simulink model "Sim2dot0"  (R2023b)
settings: Solver=VariableStepAuto  StartTime=0.0  StopTime=8  RelTol=1e-3
values from neighbouring files (symbols this model uses):
  cg_z = 0.335    [para_sim1dot4.mat]    (also in para_sim1dot5.mat; para_sim1dot6.mat = 0.215; para_sim1dot7.mat = 0.215)
  dt = 0.02    [para_sim1dot0.mat]    (also in para_sim1dot1.mat; para_sim1dot2.mat; para_sim1dot3.mat; para_sim1dot4.mat)
  F35thrust = [0 0.011 0.018 0.024 0.031 0.037 0.046 0.053 0.061 0.07 0.079 0.088 ... (170 elements, 85x2)]    [para_sim1dot3.mat]    (also in para_sim1dot4.mat; para_sim1dot5.mat; para_sim1dot6.mat; para_sim1dot7.mat)
  fin_drag_over_v2 = [-30 -25 -20 -15 -10 -5 0 5 10 15 20 25 ... (26 elements, 13x2)]    [para_sim1dot2.mat]    (also in para_sim1dot3.mat; para_sim1dot4.mat; para_sim1dot5.mat; para_sim1dot6.mat)
  fin_lift_over_v2 = [-30 -25 -20 -15 -10 -5 0 5 10 15 20 25 ... (26 elements, 13x2)]    [para_sim1dot2.mat]    (also in para_sim1dot3.mat; para_sim1dot4.mat; para_sim1dot5.mat; para_sim1dot6.mat)
  l_arm_moment = 0.5    [para_sim1dot2.mat]    (also in para_sim1dot3.mat; para_sim1dot4.mat = 0.3; para_sim1dot5.mat = 0.3; para_sim1dot6.mat = 0.175)
  mass = 1    [para_sim1dot0.mat]    (also in para_sim1dot1.mat; para_sim1dot2.mat = 0.6; para_sim1dot3.mat = 0.8; para_sim1dot4.mat = 0.8)
  max_fin_angle_deg = 30    [para_sim1dot0.mat]    (also in para_sim1dot1.mat; para_sim1dot2.mat; para_sim1dot3.mat; para_sim1dot4.mat = 20)
  r_arm_moment = 0.05    [para_sim1dot2.mat]    (also in para_sim1dot3.mat; para_sim1dot4.mat; para_sim1dot5.mat; para_sim1dot6.mat = 0.065)
  servo_slew_radps = 31.4    [para_sim1dot4.mat]    (also in para_sim1dot5.mat = 5.23; para_sim1dot6.mat = 5.23; para_sim1dot7.mat = 5.23)
libraries: simulink_extras x13, simulink x3, slpidlib x3, shared6dof x1, aerolibanim x1, matrix_library x1, aerolibanimutils x1
settings Model: Creator=Zian Liu  LastModifiedBy=Zian Liu

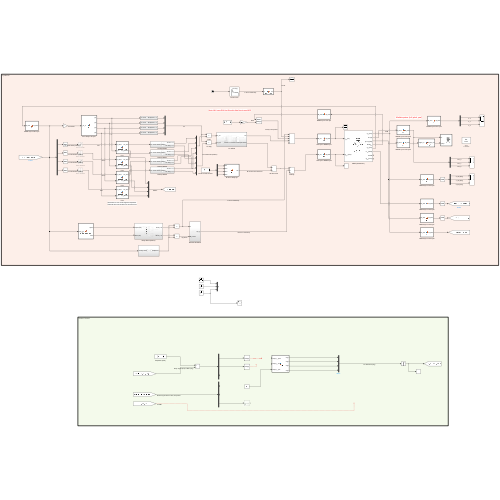
[thumbnail: Simulink's stored preview of the top-level diagram]
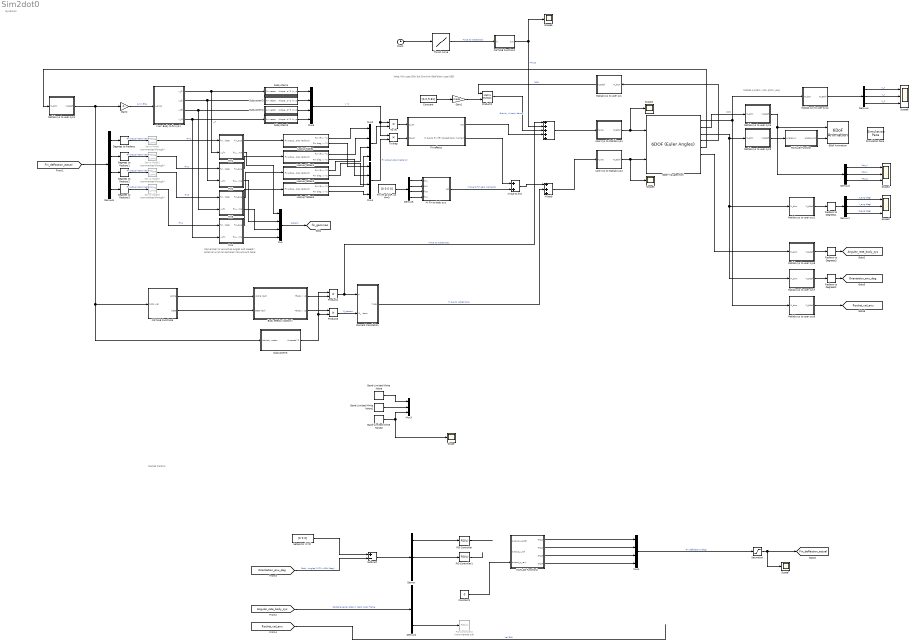
== system Sim2dot0 ==
  note: Dynamics
  note: Rocket Control
  note: Matlab system: [roll, pitch, yaw]
  note: Note: IMU uses ENU but Simulink 6dof block uses NED
  note: Remember to use actual angles and speeds!
      | External wind can be taken into account here!
  " " : Sum  Inputs=+++++
  6DOF (Quaternion) : shared6dof/6DOF (Euler Angles)  units=Metric (MKS)  mtype=Fixed  rep=Quaternion  xme_0=[0 0 0]  Vm_0=[0 0 0]  eul_0=[10*pi/180 0 0]  pm_0=[0 0 0]  mass_0=mass  mass_e=0.5  mass_f=2.0  inertia=diag([0.0301315, 0.0301315, 0.0004096])  inertia_e=eye(3)  inertia_f=2*eye(3)  k_quat=1.0  vre_flag=on  abi_flag=off  aMode=0  xme_statename=''  Vm_statename=''  eul_statename=''  quat_statename={'qr', 'qi', 'qj','qk'}  pm_statename=''  mass_statename=''
      settings: LibrarySourceBlock=aerolib6dof2/6DOF (Quaternion)
  6DoF Animation : aerolibanim/6DoF Animation  u1=[-100 100 -100 100 -300 300]  u2=0.1  u3=100  u4=[10000 0 0]  u5=Fly alongside  u6=[10000 0 0]  u7=0  u8=off
  Band-Limited White Noise : simulink/Sources/Band-Limited White Noise  Cov=[0.1]  Ts=0.01  seed=[23341]
  Band-Limited White Noise1 : simulink/Sources/Band-Limited White Noise  Cov=[0.1]  Ts=0.01  seed=[23342]
  Band-Limited White Noise2 : simulink/Sources/Band-Limited White Noise  Cov=[0.1]  Ts=0.01  seed=[23343]
  Body effects (bottom) : Subsystem
  Clock : Clock
  Constant : Constant  Value=[0,0,9.81]
  Constant1 : Constant  Value=0
  Degrees to Radians{,1..3} (4 alike) : simulink_extras/Transformations/Degrees to Radians
  Demux{,1..4} (5 alike) : Demux  Outputs=3
  Demux5 : Demux
  Demux6 : Demux
  Fin effects : Subsystem
  "Fin lift at CoP, so M=0" : Constant  Value=[0 0 0 0]
  Fin1 : MATLAB Function  TreatAsAtomicUnit=on
  Fin2 : MATLAB Function  TreatAsAtomicUnit=on
  Fin3 : MATLAB Function  TreatAsAtomicUnit=on
  Fin4 : MATLAB Function  TreatAsAtomicUnit=on
  Gain1 : Gain  Gain=mass
  Gain2 : Gain  Gain=-1
  Lookup Tables : Subsystem
  Lookup Tables1 : Subsystem
  Lookup Tables2 : Subsystem
  Lookup Tables3 : Subsystem
  M body : Sum  Inputs=+++
  M due to fins : Sum
  M: Fin to body sys : MATLAB Function  TreatAsAtomicUnit=on
  MATLAB Function : MATLAB Function  TreatAsAtomicUnit=on
  MATLAB Function1 : MATLAB Function  TreatAsAtomicUnit=on
  MATLAB Function2 : MATLAB Function  TreatAsAtomicUnit=on
  MATLAB Function6 : MATLAB Function  TreatAsAtomicUnit=on
  Matlab sys to user sys : MATLAB Function  TreatAsAtomicUnit=on
  Matlab sys to user sys1 : MATLAB Function  TreatAsAtomicUnit=on
  Matlab sys to user sys2 : MATLAB Function  TreatAsAtomicUnit=on
  Matlab sys to user sys3 : MATLAB Function  TreatAsAtomicUnit=on
  Matlab sys to user sys4 : MATLAB Function  TreatAsAtomicUnit=on
  Matlab sys to user sys5 : MATLAB Function  TreatAsAtomicUnit=on
  Matlab sys to user sys6 : MATLAB Function  TreatAsAtomicUnit=on
  Matlab sys to user sys7 : MATLAB Function  TreatAsAtomicUnit=on
  Matlab sys to user sys8 : MATLAB Function  TreatAsAtomicUnit=on
  Moment translation : Subsystem
  Mux{,1..2,4..5} (5 alike) : Mux
  Mux3 : Mux  Inputs=3
  PID Controller : slpidlib/PID Controller  Controller=PID  Form=Parallel  TimeDomain=Discrete-time  UseExternalTs=off  SampleTime=dt  IntegratorMethod=Forward Euler  FilterMethod=Forward Euler  ControllerParametersSource=internal  P=0.5  I=0  UseKiTs=off  D=0  N=100  UseFilter=on  TunerSelectOption=Transfer Function Based (PID Tuner App)  InitialConditionSource=internal  InitialConditionForIntegrator=0  InitialConditionForFilter=0  DifferentiatorICPrevScaledInput=0  ExternalReset=none  TrackingMode=off  Kt=1  LimitOutput=off  SatLimitsSource=internal  UpperSaturationLimit=inf  LowerSaturationLimit=-inf  LinearizeAsGain=on  AntiWindupMode=none  Kb=1  LimitIntegrator=off  UpperIntegratorSaturationLimit=inf  LowerIntegratorSaturationLimit=-inf  POutMin=[]  POutMax=[]  IOutMin=[]  IOutMax=[]  DOutMin=[]  DOutMax=[]  NOutMin=[]  NOutMax=[]  SumOutMin=[]  SumOutMax=[]  SaturationOutMin=[]  SaturationOutMax=[]  PParamMin=[]  PParamMax=[]  IParamMin=[]  IParamMax=[]  DParamMin=[]  DParamMax=[]  NParamMin=[]  NParamMax=[]  KbParamMin=[]  KbParamMax=[]  KtParamMin=[]  KtParamMax=[]  KbOutMin=[]  KbOutMax=[]  KtOutMin=[]  KtOutMax=[]  IntegratorOutMin=[]  IntegratorOutMax=[]  FilterOutMin=[]  FilterOutMax=[]  SumI1OutMin=[]  SumI1OutMax=[]  SumI2OutMin=[]  SumI2OutMax=[]  SumI3OutMin=[]  SumI3OutMax=[]  SumI4OutMin=[]  SumI4OutMax=[]  SumDOutMin=[]  SumDOutMax=[]  DifferentiatorOutMin=[]  DifferentiatorOutMax=[]  FilterDiffOutCoefMin=[]  FilterDiffOutCoefMax=[]  ReciprocalOutMin=[]  ReciprocalOutMax=[]  SumDenOutMin=[]  SumDenOutMax=[]  SumNumOutMin=[]  SumNumOutMax=[]  DivideOutMin=[]  DivideOutMax=[]  UdiffTsProdOutMin=[]  UdiffTsProdOutMax=[]  NTsProdOutMin=[]  NTsProdOutMax=[]  UintegralTsProdOutMin=[]  UintegralTsProdOutMax=[]  UngainTsProdOutMin=[]  UngainTsProdOutMax=[]  ClampingZeroOutDataTypeStr=Inherit: Inherit via back propagation  ClampingZeroOutMin=[]  ClampingZeroOutMax=[]  FilterDenConstantOutDataTypeStr=Inherit: Inherit via back propagation  FilterDenConstantOutMin=[]  FilterDenConstantOutMax=[]  PCopyOutDataTypeStr=Inherit: Inherit via back propagation  PCopyOutMin=[]  PCopyOutMax=[]  NCopyOutDataTypeStr=Inherit: Inherit via back propagation  NCopyOutMin=[]  NCopyOutMax=[]  IntegratorContinuousStateAttributes=''  IntegratorStateMustResolveToSignalObject=off  IntegratorRTWStateStorageClass=Auto  FilterContinuousStateAttributes=''  FilterStateMustResolveToSignalObject=off  FilterRTWStateStorageClass=Auto  ParallelPVariant=InternalParameters  IdealPVariant=Disabled  IVariant=InternalParameters  DVariant=InternalParameters  IntegratorVariant=Discrete  SatVariant=Disabled  AWVariant=Passthrough  PCopyVariant=Disabled  TRVariant=Disabled  FdbkBlocksVariant=Forward  IdealPFdbkVariant=Disabled  SatFdbkVariant=Disabled  DerivativeFilterVariant=ForwardEulerFilter  NVariant=InternalParameters  NCopyVariant=Disabled  FilterICVariant=InternalICsFilter  IntegratorICVariant=InternalICs  ExternalResetVariant=Disabled  TRSumVariant=Passthrough  SumFdbkVariant=Disabled  SumVariant=Sum_PID  TsampFilterVariant=InternalTs  TsampNgainVariant=Passthrough  TsampIntegralVariant=Disabled_SignalSpec  ExternalSaturationOutDataTypeStr=Inherit: Same as second input
  PID Controller1 : slpidlib/PID Controller  Controller=PID  Form=Parallel  TimeDomain=Discrete-time  UseExternalTs=off  SampleTime=dt  IntegratorMethod=Forward Euler  FilterMethod=Forward Euler  ControllerParametersSource=internal  P=0.5  I=0  UseKiTs=off  D=0  N=100  UseFilter=on  TunerSelectOption=Transfer Function Based (PID Tuner App)  InitialConditionSource=internal  InitialConditionForIntegrator=0  InitialConditionForFilter=0  DifferentiatorICPrevScaledInput=0  ExternalReset=none  TrackingMode=off  Kt=1  LimitOutput=off  SatLimitsSource=internal  UpperSaturationLimit=inf  LowerSaturationLimit=-inf  LinearizeAsGain=on  AntiWindupMode=none  Kb=1  LimitIntegrator=off  UpperIntegratorSaturationLimit=inf  LowerIntegratorSaturationLimit=-inf  POutMin=[]  POutMax=[]  IOutMin=[]  IOutMax=[]  DOutMin=[]  DOutMax=[]  NOutMin=[]  NOutMax=[]  SumOutMin=[]  SumOutMax=[]  SaturationOutMin=[]  SaturationOutMax=[]  PParamMin=[]  PParamMax=[]  IParamMin=[]  IParamMax=[]  DParamMin=[]  DParamMax=[]  NParamMin=[]  NParamMax=[]  KbParamMin=[]  KbParamMax=[]  KtParamMin=[]  KtParamMax=[]  KbOutMin=[]  KbOutMax=[]  KtOutMin=[]  KtOutMax=[]  IntegratorOutMin=[]  IntegratorOutMax=[]  FilterOutMin=[]  FilterOutMax=[]  SumI1OutMin=[]  SumI1OutMax=[]  SumI2OutMin=[]  SumI2OutMax=[]  SumI3OutMin=[]  SumI3OutMax=[]  SumI4OutMin=[]  SumI4OutMax=[]  SumDOutMin=[]  SumDOutMax=[]  DifferentiatorOutMin=[]  DifferentiatorOutMax=[]  FilterDiffOutCoefMin=[]  FilterDiffOutCoefMax=[]  ReciprocalOutMin=[]  ReciprocalOutMax=[]  SumDenOutMin=[]  SumDenOutMax=[]  SumNumOutMin=[]  SumNumOutMax=[]  DivideOutMin=[]  DivideOutMax=[]  UdiffTsProdOutMin=[]  UdiffTsProdOutMax=[]  NTsProdOutMin=[]  NTsProdOutMax=[]  UintegralTsProdOutMin=[]  UintegralTsProdOutMax=[]  UngainTsProdOutMin=[]  UngainTsProdOutMax=[]  ClampingZeroOutDataTypeStr=Inherit: Inherit via back propagation  ClampingZeroOutMin=[]  ClampingZeroOutMax=[]  FilterDenConstantOutDataTypeStr=Inherit: Inherit via back propagation  FilterDenConstantOutMin=[]  FilterDenConstantOutMax=[]  PCopyOutDataTypeStr=Inherit: Inherit via back propagation  PCopyOutMin=[]  PCopyOutMax=[]  NCopyOutDataTypeStr=Inherit: Inherit via back propagation  NCopyOutMin=[]  NCopyOutMax=[]  IntegratorContinuousStateAttributes=''  IntegratorStateMustResolveToSignalObject=off  IntegratorRTWStateStorageClass=Auto  FilterContinuousStateAttributes=''  FilterStateMustResolveToSignalObject=off  FilterRTWStateStorageClass=Auto  ParallelPVariant=InternalParameters  IdealPVariant=Disabled  IVariant=InternalParameters  DVariant=InternalParameters  IntegratorVariant=Discrete  SatVariant=Disabled  AWVariant=Passthrough  PCopyVariant=Disabled  TRVariant=Disabled  FdbkBlocksVariant=Forward  IdealPFdbkVariant=Disabled  SatFdbkVariant=Disabled  DerivativeFilterVariant=ForwardEulerFilter  NVariant=InternalParameters  NCopyVariant=Disabled  FilterICVariant=InternalICsFilter  IntegratorICVariant=InternalICs  ExternalResetVariant=Disabled  TRSumVariant=Passthrough  SumFdbkVariant=Disabled  SumVariant=Sum_PID  TsampFilterVariant=InternalTs  TsampNgainVariant=Passthrough  TsampIntegralVariant=Disabled_SignalSpec  ExternalSaturationOutDataTypeStr=Inherit: Same as second input
  PID Controller2 : slpidlib/PID Controller  Commented=on  Controller=PID  Form=Parallel  TimeDomain=Discrete-time  UseExternalTs=off  SampleTime=dt  IntegratorMethod=Forward Euler  FilterMethod=Forward Euler  ControllerParametersSource=internal  P=-0.1  I=0  UseKiTs=off  D=0  N=100  UseFilter=on  TunerSelectOption=Transfer Function Based (PID Tuner App)  InitialConditionSource=internal  InitialConditionForIntegrator=0  InitialConditionForFilter=0  DifferentiatorICPrevScaledInput=0  ExternalReset=none  TrackingMode=off  Kt=1  LimitOutput=off  SatLimitsSource=internal  UpperSaturationLimit=inf  LowerSaturationLimit=-inf  LinearizeAsGain=on  AntiWindupMode=none  Kb=1  LimitIntegrator=off  UpperIntegratorSaturationLimit=inf  LowerIntegratorSaturationLimit=-inf  POutMin=[]  POutMax=[]  IOutMin=[]  IOutMax=[]  DOutMin=[]  DOutMax=[]  NOutMin=[]  NOutMax=[]  SumOutMin=[]  SumOutMax=[]  SaturationOutMin=[]  SaturationOutMax=[]  PParamMin=[]  PParamMax=[]  IParamMin=[]  IParamMax=[]  DParamMin=[]  DParamMax=[]  NParamMin=[]  NParamMax=[]  KbParamMin=[]  KbParamMax=[]  KtParamMin=[]  KtParamMax=[]  KbOutMin=[]  KbOutMax=[]  KtOutMin=[]  KtOutMax=[]  IntegratorOutMin=[]  IntegratorOutMax=[]  FilterOutMin=[]  FilterOutMax=[]  SumI1OutMin=[]  SumI1OutMax=[]  SumI2OutMin=[]  SumI2OutMax=[]  SumI3OutMin=[]  SumI3OutMax=[]  SumI4OutMin=[]  SumI4OutMax=[]  SumDOutMin=[]  SumDOutMax=[]  DifferentiatorOutMin=[]  DifferentiatorOutMax=[]  FilterDiffOutCoefMin=[]  FilterDiffOutCoefMax=[]  ReciprocalOutMin=[]  ReciprocalOutMax=[]  SumDenOutMin=[]  SumDenOutMax=[]  SumNumOutMin=[]  SumNumOutMax=[]  DivideOutMin=[]  DivideOutMax=[]  UdiffTsProdOutMin=[]  UdiffTsProdOutMax=[]  NTsProdOutMin=[]  NTsProdOutMax=[]  UintegralTsProdOutMin=[]  UintegralTsProdOutMax=[]  UngainTsProdOutMin=[]  UngainTsProdOutMax=[]  ClampingZeroOutDataTypeStr=Inherit: Inherit via back propagation  ClampingZeroOutMin=[]  ClampingZeroOutMax=[]  FilterDenConstantOutDataTypeStr=Inherit: Inherit via back propagation  FilterDenConstantOutMin=[]  FilterDenConstantOutMax=[]  PCopyOutDataTypeStr=Inherit: Inherit via back propagation  PCopyOutMin=[]  PCopyOutMax=[]  NCopyOutDataTypeStr=Inherit: Inherit via back propagation  NCopyOutMin=[]  NCopyOutMax=[]  IntegratorContinuousStateAttributes=''  IntegratorStateMustResolveToSignalObject=off  IntegratorRTWStateStorageClass=Auto  FilterContinuousStateAttributes=''  FilterStateMustResolveToSignalObject=off  FilterRTWStateStorageClass=Auto  ParallelPVariant=InternalParameters  IdealPVariant=Disabled  IVariant=InternalParameters  DVariant=InternalParameters  IntegratorVariant=Discrete  SatVariant=Disabled  AWVariant=Passthrough  PCopyVariant=Disabled  TRVariant=Disabled  FdbkBlocksVariant=Forward  IdealPFdbkVariant=Disabled  SatFdbkVariant=Disabled  DerivativeFilterVariant=ForwardEulerFilter  NVariant=InternalParameters  NCopyVariant=Disabled  FilterICVariant=InternalICsFilter  IntegratorICVariant=InternalICs  ExternalResetVariant=Disabled  TRSumVariant=Passthrough  SumFdbkVariant=Disabled  SumVariant=Sum_PID  TsampFilterVariant=InternalTs  TsampNgainVariant=Passthrough  TsampIntegralVariant=Disabled_SignalSpec  ExternalSaturationOutDataTypeStr=Inherit: Same as second input
  Product1 : Product
  Product2 : Product  Multiplication=Matrix(*)
  Product3 : Product
  Radians to Degrees1 : simulink_extras/Transformations/Radians to Degrees
  Radians to Degrees2 : simulink_extras/Transformations/Radians to Degrees
  Radians to Degrees3 : simulink_extras/Transformations/Radians to Degrees
  Saturation : Saturate  UpperLimit=max_fin_angle_deg  LowerLimit=-max_fin_angle_deg
  Scope{,1,3,5,7} (5 alike) : Scope
  Scope2 : Scope  NumInputPorts=3
  Scope4 : Scope  NumInputPorts=3
  Scope6 : Scope  NumInputPorts=3
  Servo Model{,1..3} (4 alike) : RateLimiter  Commented=through  RisingSlewLimit=servo_slew_radps  FallingSlewLimit=-servo_slew_radps  SampleTimeMode=inherited
  Setpoints (XYZ) : Constant  Value=[0 0 0]
  Simulation Pace : aerolibanimutils/Simulation Pace  SimulationPace=1  SleepMode=Auto  OutputPaceError=off  SampleTime=1/30
  Subsystem1 : Subsystem
  Subsystem2 : Subsystem
  Subsystem3 : Subsystem
  Subsystem4 : Subsystem
  Subsystem5 : Subsystem
  Subtract : Sum  Inputs=+-
  Thrust curve : Lookup_n-D  NumberOfTableDimensions=1  BreakpointsForDimension1=F35thrust(:,1)  Table=F35thrust(:,2)  ExtrapMethod=Clip  InternalRulePriority=Speed  RndMeth=Simplest
  To drag : Product
  To lift : Product
  User sys to Matlab sys1 : MATLAB Function  TreatAsAtomicUnit=on
  User sys to Matlab sys2 : MATLAB Function  TreatAsAtomicUnit=on
  V air: Body to fin sys1 : MATLAB Function  TreatAsAtomicUnit=on
  tag scope: Angular_rate_body_sys=global, Fin_deflection_actual=global, Orientation_enu_deg=global, Rocket_vel_enu=global, fin_gammas=global
  wires:
  [Orientation_enu_deg] -> Subtract/2  "Body: Angles (XYZ) in ENU (deg)"
  Setpoints (XYZ)/1 -> Subtract/1
  Mux1/1 -> Saturation/1  "Fin deflections (deg)"
  Saturation/1 -> Scope7/1, [Fin_deflection_actual]
  Fin1/2(fin_gamma) -> Mux/1
  Subsystem4/1(Airspeed^2 in yz) -> Mux5/1
  Mux/1 -> [fin_gammas]  "radians"
  Demux5/4 -> M: Fin to body sys/4(fin4)
  To drag/1 -> Fin effects/2(cd_arr)
  Demux1/3 -> Scope2/3  "Z_ang (deg)"
  User sys to Matlab sys1/1(M_6dof) -> 6DOF (Quaternion)/1, Scope1/1
  V air: Body to fin sys1/1(v_f1) -> Subsystem4/1(Air vector), Fin1/2(v_fin)  "v_f"
  MATLAB Function6/1(alpha) -> Body effects (bottom)/1(Alpha (rad))
  Moment translation/1(M_cg) -> M body/2  "M due to rocket body"
  Fin2/1(fin_aoa) -> Lookup Tables1/1(Fin actual AOAs (radians))
  "Fin lift at CoP, so M=0"/1 -> Demux5/1
  Demux1/2 -> Scope2/2  "Y_ang (deg)"
  M: Fin to body sys/1(vec) -> M due to fins/2  "M due to fin aero moments"
  Demux3/3 -> Scope4/3  "Pos_Z"
  M due to fins/1 -> M body/1
  Thrust curve/1 -> MATLAB Function1/1(in)  "F due to rocket body"
  Demux5/1 -> M: Fin to body sys/1(fin1)
  Demux5/2 -> M: Fin to body sys/2(fin2)
  MATLAB Function/1(angles_out) -> 6DoF Animation/2
  Matlab sys to user sys5/1(M_6dof) -> Demux3/1, 6DoF Animation/1
  M body/1 -> User sys to Matlab sys2/1(M_me)
  6DOF (Quaternion)/2 -> Matlab sys to user sys5/1(M_dcm)  "DCM"
  Subsystem2/1(Airspeed^2 in yz) -> Mux5/2
  V air: Body to fin sys1/3(v_f3) -> Subsystem1/1(Air vector), Fin3/2(v_fin)
  MATLAB Function1/1(out) -> Scope5/1, " "/2  "Thrust"
  Product2/1 -> " "/3  "Gravity in body frame"
  Matlab sys to user sys3/1(M_6dof) -> MATLAB Function/1(angles_in)
  Gain2/1 -> V air: Body to fin sys1/1(v_air_b)  "Air in ENU"
  Gain1/1 -> Product2/2
  Subsystem3/1(Airspeed^2 in yz) -> Mux5/4
  Matlab sys to user sys1/1(M_6dof) -> Subsystem5/1(Velocity vector), MATLAB Function6/1(body_vel), Gain2/1
  Mux2/1 -> To lift/2
  Demux3/2 -> Scope4/2  "Pos_Y"
  " "/1 -> User sys to Matlab sys1/1(M_me)
  Constant/1 -> Gain1/1
  6DOF (Quaternion)/3 -> Matlab sys to user sys7/1(M_dcm), Matlab sys to user sys2/1(M_dcm), Matlab sys to user sys3/1(M_dcm)
  Demux6/1 -> Degrees to Radians/1
  Subsystem1/1(Airspeed^2 in yz) -> Mux5/3
  User sys to Matlab sys2/1(M_6dof) -> Scope3/1, 6DOF (Quaternion)/2
  Subsystem5/1(Airspeed^2) -> Product1/1, Product3/2
  Mux5/1 -> To drag/1, To lift/1  "v^2"
  MATLAB Function6/2(beta) -> Body effects (bottom)/2(Beta (rad))
  Product3/1 -> Moment translation/2(M_bottom)  "M_bottom"
  Product1/1 -> Moment translation/1(F), " "/1  "F due to rocket body"
  Lookup Tables/2(Fin drag / v^2) -> Mux4/1
  Body effects (bottom)/2(Mbody / v2) -> Product3/1
  Matlab sys to user sys2/1(M_6dof) -> Radians to Degrees1/1
  Matlab sys to user sys4/1(M_6dof) -> Demux4/1
  Lookup Tables1/2(Fin drag / v^2) -> Mux4/2
  V air: Body to fin sys1/2(v_f2) -> Subsystem2/1(Air vector), Fin2/2(v_fin)
  Radians to Degrees1/1 -> Demux1/1
  Band-Limited White Noise2/1 -> Scope/1, Mux3/3
  Fin1/1(fin_aoa) -> Lookup Tables/1(Fin actual AOAs (radians))
  Lookup Tables3/2(Fin drag / v^2) -> Mux4/4
  Band-Limited White Noise1/1 -> Mux3/2
  Lookup Tables2/1(Fin lift / v^2) -> Mux2/3
  Fin effects/2(M due to fin lift induced body moments) -> M due to fins/1
  Fin3/2(fin_gamma) -> Mux/3
  V air: Body to fin sys1/4(v_f4) -> Subsystem3/1(Air vector), Fin4/2(v_fin)
  Clock/1 -> Thrust curve/1
  Demux1/1 -> Scope2/1  "X_ang (deg)"
  6DOF (Quaternion)/4 -> Matlab sys to user sys/1(M_dcm)
  To lift/1 -> Fin effects/1(cl_arr)
  Mux4/1 -> To drag/2  "Fin actual AOAs (radians)"
  Demux3/1 -> Scope4/1  "Pos_X"
  Servo Model/1 -> Fin1/1(fin_theta)  "Fin1"
  Fin2/2(fin_gamma) -> Mux/2
  6DOF (Quaternion)/5 -> Matlab sys to user sys1/1(M_dcm)
  Fin3/1(fin_aoa) -> Lookup Tables2/1(Fin actual AOAs (radians))
  Body effects (bottom)/1(Fbody / v2) -> Product1/2
  Matlab sys to user sys/1(M_6dof) -> Product2/1  "DCM"
  Lookup Tables2/2(Fin drag / v^2) -> Mux4/3
  Fin4/1(fin_aoa) -> Lookup Tables3/1(Fin actual AOAs (radians))
  Demux4/3 -> Scope6/3  "V_Z"
  Band-Limited White Noise/1 -> Mux3/1
  Lookup Tables3/1(Fin lift / v^2) -> Mux2/4
  Lookup Tables/1(Fin lift / v^2) -> Mux2/1
  Fin effects/1(vec) -> " "/4
  Lookup Tables1/1(Fin lift / v^2) -> Mux2/2
  Demux5/3 -> M: Fin to body sys/3(fin3)
  Fin4/2(fin_gamma) -> Mux/4
  Demux4/2 -> Scope6/2  "V_Y"
  Demux4/1 -> Scope6/1  "V_X"
  Degrees to Radians/1 -> Servo Model/1  "Fin actual AOAs (radians)"
  6DOF (Quaternion)/6 -> Matlab sys to user sys6/1(M_dcm)
  Matlab sys to user sys6/1(M_6dof) -> Radians to Degrees3/1
  Matlab sys to user sys7/1(M_6dof) -> Radians to Degrees2/1
  Radians to Degrees2/1 -> [Orientation_enu_deg]
  Radians to Degrees3/1 -> [Angular_rate_body_sys]
  6DOF (Quaternion)/1 -> Matlab sys to user sys8/1(M_dcm), Matlab sys to user sys4/1(M_dcm)
  Matlab sys to user sys8/1(M_6dof) -> [Rocket_vel_enu]
  [Fin_deflection_actual] -> Demux6/1
  Demux6/2 -> Degrees to Radians1/1
  Degrees to Radians1/1 -> Servo Model1/1  "Fin actual AOAs (radians)"
  Servo Model1/1 -> Fin2/1(fin_theta)  "Fin2"
  Demux6/3 -> Degrees to Radians2/1
  Degrees to Radians2/1 -> Servo Model2/1  "Fin actual AOAs (radians)"
  Servo Model2/1 -> Fin3/1(fin_theta)  "Fin3"
  Demux6/4 -> Degrees to Radians3/1
  Degrees to Radians3/1 -> Servo Model3/1  "Fin actual AOAs (radians)"
  Servo Model3/1 -> Fin4/1(fin_theta)  "Fin4"
  Subtract/1 -> Demux/1
  Demux/1 -> PID Controller/1
  MATLAB Function2/1(ang1) -> Mux1/1
  MATLAB Function2/2(ang2) -> Mux1/2
  MATLAB Function2/3(ang3) -> Mux1/3
  MATLAB Function2/4(ang4) -> Mux1/4
  Demux/2 -> PID Controller1/1
  [Rocket_vel_enu] -> ?  "Vel ENU"
  Demux2/3 -> PID Controller2/1
  Constant1/1 -> MATLAB Function2/3(output_z_yaw)
  [Angular_rate_body_sys] -> Demux2/1  "Rocket angular rates in rad/s, body frame"
  PID Controller/1 -> ?
  PID Controller1/1 -> ?

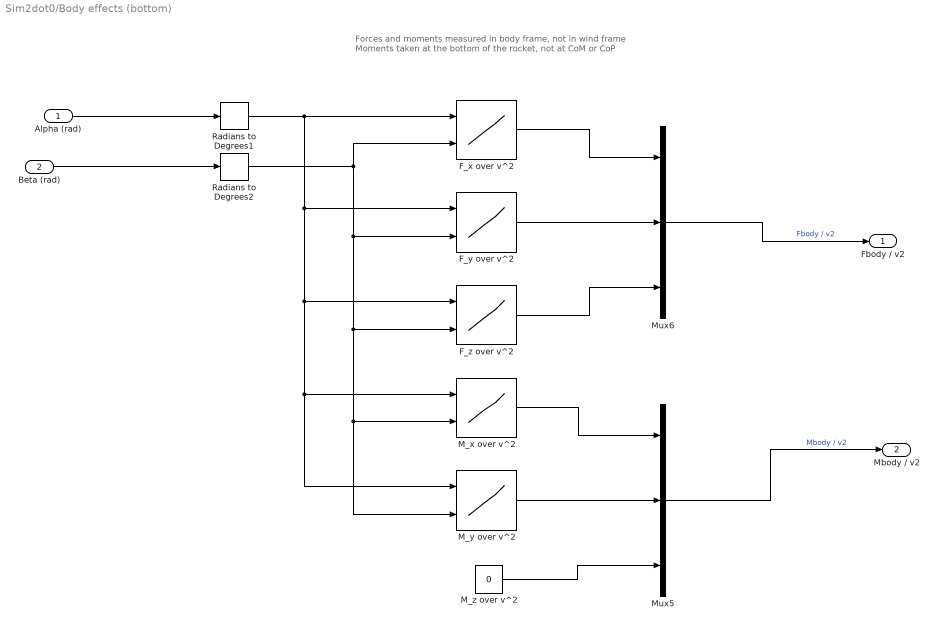
== system Sim2dot0/Body effects (bottom) ==
  note: Forces and moments measured in body frame, not in wind frame
      |
      | Moments taken at the bottom of the rocket, not at CoM or CoP
  Alpha (rad) : Inport
  Beta (rad) : Inport  Port=2
  F_x over v^2 : Lookup_n-D  BreakpointsForDimension1=body_Fx_over_v2(2:end,1)  BreakpointsForDimension2=body_Fx_over_v2(1,2:end)  BreakpointsForDimension3=[5, 7]  Table=body_Fx_over_v2(2:end,2:end)  ExtrapMethod=Clip  InternalRulePriority=Speed  RndMeth=Simplest
      settings: InputPortMap=u0,u1
  F_y over v^2 : Lookup_n-D  BreakpointsForDimension1=body_Fy_over_v2(2:end,1)  BreakpointsForDimension2=body_Fy_over_v2(1,2:end)  BreakpointsForDimension3=[5, 7]  Table=body_Fy_over_v2(2:end,2:end)  ExtrapMethod=Clip  InternalRulePriority=Speed  RndMeth=Simplest
      settings: InputPortMap=u0,u1
  F_z over v^2 : Lookup_n-D  BreakpointsForDimension1=body_Fz_over_v2(2:end,1)  BreakpointsForDimension2=body_Fz_over_v2(1,2:end)  BreakpointsForDimension3=[5, 7]  Table=body_Fz_over_v2(2:end,2:end)  ExtrapMethod=Clip  InternalRulePriority=Speed  RndMeth=Simplest
      settings: InputPortMap=u0,u1
  M_x over v^2 : Lookup_n-D  BreakpointsForDimension1=body_Mx_over_v2(2:end,1)  BreakpointsForDimension2=body_Mx_over_v2(1,2:end)  BreakpointsForDimension3=[5, 7]  Table=body_Mx_over_v2(2:end,2:end)  ExtrapMethod=Clip  InternalRulePriority=Speed  RndMeth=Simplest
      settings: InputPortMap=u0,u1
  M_y over v^2 : Lookup_n-D  BreakpointsForDimension1=body_My_over_v2(2:end,1)  BreakpointsForDimension2=body_My_over_v2(1,2:end)  BreakpointsForDimension3=[5, 7]  Table=body_My_over_v2(2:end,2:end)  ExtrapMethod=Clip  InternalRulePriority=Speed  RndMeth=Simplest
      settings: InputPortMap=u0,u1
  M_z over v^2 : Constant  Value=0
  Mux5 : Mux  Inputs=3
  Mux6 : Mux  Inputs=3
  Radians to Degrees1 : simulink_extras/Transformations/Radians to Degrees
  Radians to Degrees2 : simulink_extras/Transformations/Radians to Degrees
  Fbody / v2 : Outport
  Mbody / v2 : Outport  Port=2
  wires:
  F_y over v^2/1 -> Mux6/2
  M_x over v^2/1 -> Mux5/1
  Radians to Degrees1/1 -> M_y over v^2/1, M_x over v^2/1, F_z over v^2/1, F_y over v^2/1, F_x over v^2/1
  Radians to Degrees2/1 -> F_x over v^2/2, M_y over v^2/2, M_x over v^2/2, F_z over v^2/2, F_y over v^2/2
  F_x over v^2/1 -> Mux6/1
  Mux6/1 -> Fbody / v2/1  "Fbody / v2"
  M_y over v^2/1 -> Mux5/2
  Alpha (rad)/1 -> Radians to Degrees1/1
  M_z over v^2/1 -> Mux5/3
  F_z over v^2/1 -> Mux6/3
  Mux5/1 -> Mbody / v2/1  "Mbody / v2"
  Beta (rad)/1 -> Radians to Degrees2/1

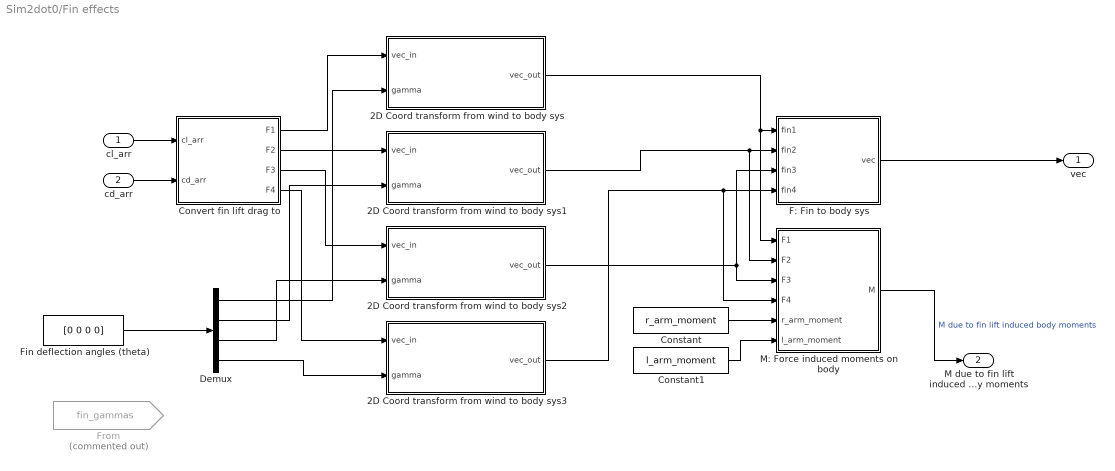
== system Sim2dot0/Fin effects ==
  cl_arr : Inport
  cd_arr : Inport  Port=2
  2D Coord transform from wind to body sys : MATLAB Function  TreatAsAtomicUnit=on
  2D Coord transform from wind to body sys1 : MATLAB Function  TreatAsAtomicUnit=on
  2D Coord transform from wind to body sys2 : MATLAB Function  TreatAsAtomicUnit=on
  2D Coord transform from wind to body sys3 : MATLAB Function  TreatAsAtomicUnit=on
  Constant : Constant  Value=r_arm_moment
  Constant1 : Constant  Value=l_arm_moment
  "Convert fin lift drag to " : MATLAB Function  TreatAsAtomicUnit=on
  Demux : Demux
  F: Fin to body sys : MATLAB Function  TreatAsAtomicUnit=on
  Fin deflection angles (theta) : Constant  Value=[0 0 0 0]
  From : From  Commented=on  GotoTag=fin_gammas  TagVisibility=global
  M: Force induced moments on body : MATLAB Function  TreatAsAtomicUnit=on
  vec : Outport
  M due to fin lift induced body moments : Outport  Port=2
  wires:
  2D Coord transform from wind to body sys/1(vec_out) -> M: Force induced moments on body/1(F1), F: Fin to body sys/1(fin1)
  2D Coord transform from wind to body sys2/1(vec_out) -> F: Fin to body sys/3(fin3), M: Force induced moments on body/3(F3)
  2D Coord transform from wind to body sys3/1(vec_out) -> M: Force induced moments on body/4(F4), F: Fin to body sys/4(fin4)
  cl_arr/1 -> "Convert fin lift drag to "/1(cl_arr)
  2D Coord transform from wind to body sys1/1(vec_out) -> M: Force induced moments on body/2(F2), F: Fin to body sys/2(fin2)
  F: Fin to body sys/1(vec) -> vec/1
  M: Force induced moments on body/1(M) -> M due to fin lift induced body moments/1  "M due to fin lift induced body moments"
  cd_arr/1 -> "Convert fin lift drag to "/2(cd_arr)
  "Convert fin lift drag to "/1(F1) -> 2D Coord transform from wind to body sys/1(vec_in)
  "Convert fin lift drag to "/2(F2) -> 2D Coord transform from wind to body sys1/1(vec_in)
  "Convert fin lift drag to "/3(F3) -> 2D Coord transform from wind to body sys2/1(vec_in)
  "Convert fin lift drag to "/4(F4) -> 2D Coord transform from wind to body sys3/1(vec_in)
  Fin deflection angles (theta)/1 -> Demux/1
  Demux/4 -> 2D Coord transform from wind to body sys3/2(gamma)
  Demux/3 -> 2D Coord transform from wind to body sys2/2(gamma)
  Demux/2 -> 2D Coord transform from wind to body sys1/2(gamma)
  Demux/1 -> 2D Coord transform from wind to body sys/2(gamma)
  Constant/1 -> M: Force induced moments on body/5(r_arm_moment)
  Constant1/1 -> M: Force induced moments on body/6(l_arm_moment)

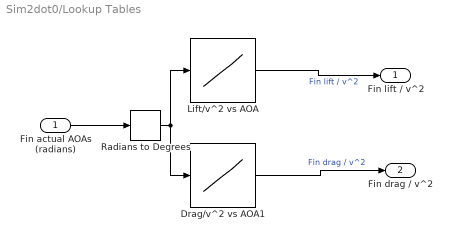
== system Sim2dot0/Lookup Tables ==
  Fin actual AOAs (radians) : Inport
  Drag/v^2 vs AOA1 : Lookup_n-D  NumberOfTableDimensions=1  BreakpointsForDimension1=fin_drag_over_v2(:,1)  Table=fin_drag_over_v2(:,2)  ExtrapMethod=Clip  InternalRulePriority=Speed  RndMeth=Simplest
  Lift/v^2 vs AOA : Lookup_n-D  NumberOfTableDimensions=1  BreakpointsForDimension1=fin_lift_over_v2(:,1)  Table=fin_lift_over_v2(:,2)  ExtrapMethod=Clip  InternalRulePriority=Speed  RndMeth=Simplest
  Radians to Degrees : simulink_extras/Transformations/Radians to Degrees
  Fin lift / v^2 : Outport
  Fin drag / v^2 : Outport  Port=2
  wires:
  Radians to Degrees/1 -> Lift/v^2 vs AOA/1, Drag/v^2 vs AOA1/1
  Drag/v^2 vs AOA1/1 -> Fin drag / v^2/1  "Fin drag / v^2"
  Lift/v^2 vs AOA/1 -> Fin lift / v^2/1  "Fin lift / v^2"
  Fin actual AOAs (radians)/1 -> Radians to Degrees/1

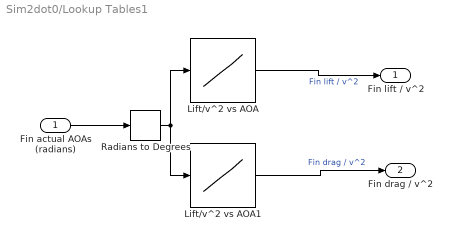
== system Sim2dot0/Lookup Tables1 ==
  Fin actual AOAs (radians) : Inport
  Lift/v^2 vs AOA : Lookup_n-D  NumberOfTableDimensions=1  BreakpointsForDimension1=fin_lift_over_v2(:,1)  Table=fin_lift_over_v2(:,2)  ExtrapMethod=Clip  InternalRulePriority=Speed  RndMeth=Simplest
  Lift/v^2 vs AOA1 : Lookup_n-D  NumberOfTableDimensions=1  BreakpointsForDimension1=fin_drag_over_v2(:,1)  Table=fin_drag_over_v2(:,2)  ExtrapMethod=Clip  InternalRulePriority=Speed  RndMeth=Simplest
  Radians to Degrees : simulink_extras/Transformations/Radians to Degrees
  Fin lift / v^2 : Outport
  Fin drag / v^2 : Outport  Port=2
  wires:
  Radians to Degrees/1 -> Lift/v^2 vs AOA/1, Lift/v^2 vs AOA1/1
  Lift/v^2 vs AOA1/1 -> Fin drag / v^2/1  "Fin drag / v^2"
  Lift/v^2 vs AOA/1 -> Fin lift / v^2/1  "Fin lift / v^2"
  Fin actual AOAs (radians)/1 -> Radians to Degrees/1

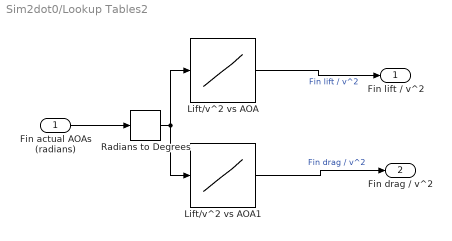
== system Sim2dot0/Lookup Tables2 ==
  Fin actual AOAs (radians) : Inport
  Lift/v^2 vs AOA : Lookup_n-D  NumberOfTableDimensions=1  BreakpointsForDimension1=fin_lift_over_v2(:,1)  Table=fin_lift_over_v2(:,2)  ExtrapMethod=Clip  InternalRulePriority=Speed  RndMeth=Simplest
  Lift/v^2 vs AOA1 : Lookup_n-D  NumberOfTableDimensions=1  BreakpointsForDimension1=fin_drag_over_v2(:,1)  Table=fin_drag_over_v2(:,2)  ExtrapMethod=Clip  InternalRulePriority=Speed  RndMeth=Simplest
  Radians to Degrees : simulink_extras/Transformations/Radians to Degrees
  Fin lift / v^2 : Outport
  Fin drag / v^2 : Outport  Port=2
  wires:
  Radians to Degrees/1 -> Lift/v^2 vs AOA/1, Lift/v^2 vs AOA1/1
  Lift/v^2 vs AOA1/1 -> Fin drag / v^2/1  "Fin drag / v^2"
  Lift/v^2 vs AOA/1 -> Fin lift / v^2/1  "Fin lift / v^2"
  Fin actual AOAs (radians)/1 -> Radians to Degrees/1

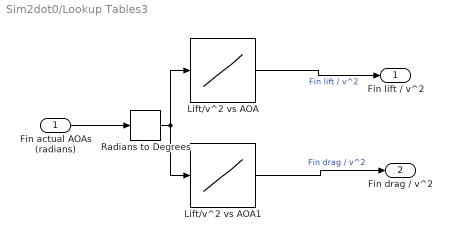
== system Sim2dot0/Lookup Tables3 ==
  Fin actual AOAs (radians) : Inport
  Lift/v^2 vs AOA : Lookup_n-D  NumberOfTableDimensions=1  BreakpointsForDimension1=fin_lift_over_v2(:,1)  Table=fin_lift_over_v2(:,2)  ExtrapMethod=Clip  InternalRulePriority=Speed  RndMeth=Simplest
  Lift/v^2 vs AOA1 : Lookup_n-D  NumberOfTableDimensions=1  BreakpointsForDimension1=fin_drag_over_v2(:,1)  Table=fin_drag_over_v2(:,2)  ExtrapMethod=Clip  InternalRulePriority=Speed  RndMeth=Simplest
  Radians to Degrees : simulink_extras/Transformations/Radians to Degrees
  Fin lift / v^2 : Outport
  Fin drag / v^2 : Outport  Port=2
  wires:
  Radians to Degrees/1 -> Lift/v^2 vs AOA/1, Lift/v^2 vs AOA1/1
  Lift/v^2 vs AOA1/1 -> Fin drag / v^2/1  "Fin drag / v^2"
  Lift/v^2 vs AOA/1 -> Fin lift / v^2/1  "Fin lift / v^2"
  Fin actual AOAs (radians)/1 -> Radians to Degrees/1

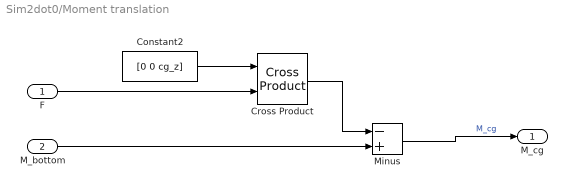
== system Sim2dot0/Moment translation ==
  F : Inport
  M_bottom : Inport  Port=2
  Constant2 : Constant  Value=[0 0 cg_z]
  Cross Product : matrix_library/Cross Product
  Minus : Sum  Inputs=-+
  M_cg : Outport
  wires:
  F/1 -> Cross Product/2
  Cross Product/1 -> Minus/1
  Constant2/1 -> Cross Product/1
  Minus/1 -> M_cg/1  "M_cg"
  M_bottom/1 -> Minus/2

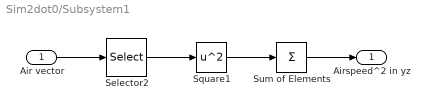
== system Sim2dot0/Subsystem1 ==
  Air vector : Inport
  Selector2 : Selector  InputPortWidth=3  IndexOptions=Index vector (dialog)  Indices=[2 3]  OutputSizes=1
  Square1 : Math  Operator=square
  Sum of Elements : Sum  Inputs=+
  Airspeed^2 in yz : Outport
  wires:
  Square1/1 -> Sum of Elements/1
  Selector2/1 -> Square1/1
  Sum of Elements/1 -> Airspeed^2 in yz/1
  Air vector/1 -> Selector2/1

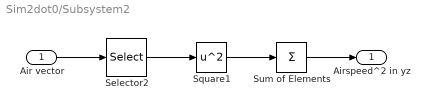
== system Sim2dot0/Subsystem2 ==
  Air vector : Inport
  Selector2 : Selector  InputPortWidth=3  IndexOptions=Index vector (dialog)  Indices=[2 3]  OutputSizes=1
  Square1 : Math  Operator=square
  Sum of Elements : Sum  Inputs=+
  Airspeed^2 in yz : Outport
  wires:
  Square1/1 -> Sum of Elements/1
  Selector2/1 -> Square1/1
  Sum of Elements/1 -> Airspeed^2 in yz/1
  Air vector/1 -> Selector2/1

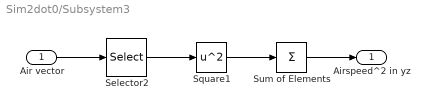
== system Sim2dot0/Subsystem3 ==
  Air vector : Inport
  Selector2 : Selector  InputPortWidth=3  IndexOptions=Index vector (dialog)  Indices=[2 3]  OutputSizes=1
  Square1 : Math  Operator=square
  Sum of Elements : Sum  Inputs=+
  Airspeed^2 in yz : Outport
  wires:
  Square1/1 -> Sum of Elements/1
  Selector2/1 -> Square1/1
  Sum of Elements/1 -> Airspeed^2 in yz/1
  Air vector/1 -> Selector2/1

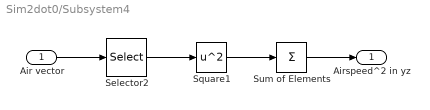
== system Sim2dot0/Subsystem4 ==
  Air vector : Inport
  Selector2 : Selector  InputPortWidth=3  IndexOptions=Index vector (dialog)  Indices=[2 3]  OutputSizes=1
  Square1 : Math  Operator=square
  Sum of Elements : Sum  Inputs=+
  Airspeed^2 in yz : Outport
  wires:
  Square1/1 -> Sum of Elements/1
  Selector2/1 -> Square1/1
  Sum of Elements/1 -> Airspeed^2 in yz/1
  Air vector/1 -> Selector2/1

== system Sim2dot0/Subsystem5 ==
  Velocity vector : Inport
  Square1 : Math  Operator=square
  Sum of Elements : Sum  Inputs=+
  Airspeed^2 : Outport
  wires:
  Square1/1 -> Sum of Elements/1
  Velocity vector/1 -> Square1/1
  Sum of Elements/1 -> Airspeed^2/1

== matlab function Sim2dot0/MATLAB Function ==
  data: angles_in input; angles_out output
function angles_out = pitchadd2pi(angles_in)
angles_out = [angles_in(1); angles_in(2)-pi/2; angles_in(3)];

== matlab function Sim2dot0/MATLAB Function1 ==
  data: in input; out output
function out = thrustz2vec(in)
out = [0 0 in];

== matlab function Sim2dot0/Matlab sys to user sys3 ==
  data: M_dcm input; M_6dof output
function M_6dof = fcn(M_dcm)
M_lab2user = [0 1 0; 1 0 0; 0 0 -1];
M_6dof = M_lab2user * M_dcm;

== matlab function Sim2dot0/Fin1 ==
  data: fin_theta input; fin_aoa output; v_fin input; fin_gamma output
function [fin_aoa, fin_gamma]= theta2aoa_fin(fin_theta, v_fin)
vz = v_fin(3);
vy = v_fin(2);
fin_gamma = - pi/2 - atan2(vz, vy); % assuming v_fin points in q3 or q4 (negative z) during launch, note vz cannot points upwards, or gamma will be big in q2
fin_aoa = fin_theta - fin_gamma;

== matlab function Sim2dot0/Matlab sys to user sys5 ==
  data: M_dcm input; M_6dof output
function M_6dof = fcn(M_dcm)
M_lab2user = [0 1 0; 1 0 0; 0 0 -1];
M_6dof = M_lab2user * M_dcm;

== matlab function Sim2dot0/Fin2 ==
  data: fin_theta input; fin_aoa output; v_fin input; fin_gamma output
function [fin_aoa, fin_gamma]= theta2aoa_fin(fin_theta, v_fin)
vz = v_fin(3);
vy = v_fin(2);
fin_gamma = - pi/2 - atan2(vz, vy); % assuming v_fin points in q3 or q4 (negative z) during launch, note vz cannot points upwards, or gamma will be big in q2
fin_aoa = fin_theta - fin_gamma;

== matlab function Sim2dot0/Fin3 ==
  data: fin_theta input; fin_aoa output; v_fin input; fin_gamma output
function [fin_aoa, fin_gamma]= theta2aoa_fin(fin_theta, v_fin)
vz = v_fin(3);
vy = v_fin(2);
fin_gamma = - pi/2 - atan2(vz, vy); % assuming v_fin points in q3 or q4 (negative z) during launch, note vz cannot points upwards, or gamma will be big in q2
fin_aoa = fin_theta - fin_gamma;

== matlab function Sim2dot0/Fin4 ==
  data: fin_theta input; fin_aoa output; v_fin input; fin_gamma output
function [fin_aoa, fin_gamma]= theta2aoa_fin(fin_theta, v_fin)
vz = v_fin(3);
vy = v_fin(2);
fin_gamma = - pi/2 - atan2(vz, vy); % assuming v_fin points in q3 or q4 (negative z) during launch, note vz cannot points upwards, or gamma will be big in q2
fin_aoa = fin_theta - fin_gamma;

== matlab function Sim2dot0/Fin effects/F: Fin to body sys ==
  data: fin1 input; vec output; fin2 input; fin3 input; fin4 input
function vec = fcn(fin1, fin2, fin3, fin4)
vx = fin1(1) - fin2(2) - fin3(1) + fin4(2);
vy = fin1(2) + fin2(1) - fin3(2) - fin4(1);
vz = fin1(3) + fin2(3) + fin3(3) + fin4(3);

vec = [vx, vy, vz];

== matlab function Sim2dot0/MATLAB Function6 ==
  data: body_vel input; alpha output; beta output
function [alpha, beta]= alpha_beta_rad(body_vel)
vt = norm(body_vel);
vx = body_vel(1);
vy = body_vel(2);
beta = asin(vx / vt);
alpha = asin(vy / (vt * cos(beta)));

== matlab function Sim2dot0/Matlab sys to user sys6 ==
  data: M_dcm input; M_6dof output
function M_6dof = fcn(M_dcm)
M_lab2user = [0 1 0; 1 0 0; 0 0 -1];
M_6dof = M_lab2user * M_dcm;

== matlab function Sim2dot0/Fin effects/2D Coord transform from wind to body sys ==
  data: vec_in input; vec_out output; gamma input
function vec_out = wind2body_fin(vec_in, gamma) % beta converts vec in wind sys to 0 fin angle sys which is parallel to rocket body sys

vec_in_T = transpose(vec_in);
vec_out = [1, 0,         0;
           0, cos(gamma), -sin(gamma);
           0, sin(gamma), cos(gamma),] * vec_in_T;

== matlab function Sim2dot0/Fin effects/2D Coord transform from wind to body sys1 ==
  data: vec_in input; vec_out output; gamma input
function vec_out = wind2body_fin(vec_in, gamma) % beta converts vec in wind sys to 0 fin angle sys which is parallel to rocket body sys

vec_in_T = transpose(vec_in);
vec_out = [1, 0,         0;
           0, cos(gamma), -sin(gamma);
           0, sin(gamma), cos(gamma),] * vec_in_T;

== matlab function Sim2dot0/Fin effects/2D Coord transform from wind to body sys2 ==
  data: vec_in input; vec_out output; gamma input
function vec_out = wind2body_fin(vec_in, gamma) % beta converts vec in wind sys to 0 fin angle sys which is parallel to rocket body sys

vec_in_T = transpose(vec_in);
vec_out = [1, 0,         0;
           0, cos(gamma), -sin(gamma);
           0, sin(gamma), cos(gamma),] * vec_in_T;

== matlab function Sim2dot0/Fin effects/2D Coord transform from wind to body sys3 ==
  data: vec_in input; vec_out output; gamma input
function vec_out = wind2body_fin(vec_in, gamma) % beta converts vec in wind sys to 0 fin angle sys which is parallel to rocket body sys

vec_in_T = transpose(vec_in);
vec_out = [1, 0,         0;
           0, cos(gamma), -sin(gamma);
           0, sin(gamma), cos(gamma),] * vec_in_T;

== matlab function Sim2dot0/Matlab sys to user sys4 ==
  data: M_dcm input; M_6dof output
function M_6dof = fcn(M_dcm)
M_lab2user = [0 1 0; 1 0 0; 0 0 -1];
M_6dof = M_lab2user * M_dcm;

== matlab function Sim2dot0/Matlab sys to user sys7 ==
  data: M_dcm input; M_6dof output
function M_6dof = fcn(M_dcm)
M_lab2user = [0 1 0; 1 0 0; 0 0 -1];
M_6dof = M_lab2user * M_dcm;

== matlab function Sim2dot0/Matlab sys to user sys8 ==
  data: M_dcm input; M_6dof output
function M_6dof = fcn(M_dcm)
M_lab2user = [0 1 0; 1 0 0; 0 0 -1];
M_6dof = M_lab2user * M_dcm;

== matlab function Sim2dot0/MATLAB Function2 ==
  data: output_x_pitch input; ang1 output; output_y_roll input; output_z_yaw input; ang2 output; ang3 output; ang4 output
function [ang1, ang2, ang3, ang4] = control2fin(output_x_pitch, output_y_roll, output_z_yaw)

ang1 = (output_z_yaw + 0. + output_x_pitch);
ang2 = (output_z_yaw + output_y_roll + 0.);
ang3 = (output_z_yaw + 0. - output_x_pitch);
ang4 = (output_z_yaw - output_y_roll + 0.);

== matlab function Sim2dot0/Matlab sys to user sys1 ==
  data: M_dcm input; M_6dof output
function M_6dof = fcn(M_dcm)
M_lab2user = [0 1 0; 1 0 0; 0 0 -1];
M_6dof = M_lab2user * M_dcm;

== matlab function Sim2dot0/M: Fin to body sys ==
  data: fin1 input; vec output; fin2 input; fin3 input; fin4 input
function vec = fcn(fin1, fin2, fin3, fin4)
vx = -fin1 + fin3; % CW moment is positive, in negative x dir
vy = -fin2 + fin4;
vz = 0;

vec = [vx, vy, vz];

== matlab function Sim2dot0/Fin effects/M: Force induced moments on body ==
  data: F1 input; M output; F2 input; F3 input; F4 input; r_arm_moment input; l_arm_moment input
function M = fcn(F1, F2, F3, F4, r_arm_moment, l_arm_moment)

r1 = [r_arm_moment, 0, -l_arm_moment];
r2 = [0, r_arm_moment, -l_arm_moment];
r3 = [-r_arm_moment, 0, -l_arm_moment];
r4 = [0, -r_arm_moment, -l_arm_moment];

F1_body = F1;
F2_body = [-F2(2) F2(1) F2(3)];
F3_body = [-F3(1) -F3(2) F3(3)];
F4_body = [F4(2) -F4(1) F4(3)];
M = cross(r1, F1_body) + cross(r2, F2_body) + cross(r3, F3_body) + cross(r4, F4_body);

== matlab function Sim2dot0/Fin effects/Convert fin lift drag to  ==
  data: cl_arr input; F1 output; cd_arr input; F2 output; F3 output; F4 output
function [F1, F2, F3, F4]= fcn(cl_arr, cd_arr)
F1 = [0, cl_arr(1), -cd_arr(1)];
F2 = [0, cl_arr(2), -cd_arr(2)];
F3 = [0, cl_arr(3), -cd_arr(3)];
F4 = [0, cl_arr(4), -cd_arr(4)];

== matlab function Sim2dot0/User sys to Matlab sys2 ==
  data: M_me input; M_6dof output
function M_6dof = fcn(M_me)
M_6dof = [M_me(2), M_me(1), -M_me(3)];

== matlab function Sim2dot0/User sys to Matlab sys1 ==
  data: M_me input; M_6dof output
function M_6dof = fcn(M_me)
M_6dof = [M_me(2), M_me(1), -M_me(3)];

== matlab function Sim2dot0/V air: Body to fin sys1 ==
  data: v_air_b input; v_f1 output; v_f2 output; v_f3 output; v_f4 output
function [v_f1, v_f2, v_f3, v_f4]= fcn(v_air_b)
vx = v_air_b(1);
vy = v_air_b(2);
vz = v_air_b(3);

v_f1 = [vx, vy, vz];
v_f2 = [vy, -vx, vz];
v_f3 = [-vx, -vy, vz];
v_f4 = [-vy, vx, vz];

== matlab function Sim2dot0/Matlab sys to user sys ==
  data: M_dcm input; M_6dof output
function M_6dof = fcn(M_dcm)
M_lab2user = [0 1 0; 1 0 0; 0 0 -1];
M_6dof = M_lab2user * M_dcm;

== matlab function Sim2dot0/Matlab sys to user sys2 ==
  data: M_dcm input; M_6dof output
function M_6dof = fcn(M_dcm)
M_lab2user = [0 1 0; 1 0 0; 0 0 -1];
M_6dof = M_lab2user * M_dcm;
